simulink model "our_ch47"  (R2021a)
settings: Solver=FixedStepAuto  StartTime=0.0  StopTime=10  FixedStep=0.001  RelTol=1e-3  AbsTol=1e-3  EnableMultiTasking=on
undefined symbols (not defined in the file or in its folder): DiscIntNeverNeededParam, e2b, envs, PID_Param1, pos1, pos2, pos3, pos4, pos_load, tandem, X, x0, Y, Z
libraries: sm_lib x88, nesl_utility x25
(part 5 of 6)

== system our_ch47/Subsystem/直升机2 PID control/姿态控制器/航向控制器H-A/Altitude_Controller ==
  YawD : Inport
  Yaw : Inport  Port=2
  Constant : Constant  Value=0  OutDataTypeStr=Inherit: Inherit via back propagation
  Controller : Subsystem
  Saturation : Saturate  UpperLimit=45  LowerLimit=-45
  Saturation1 : Saturate  UpperLimit=45  LowerLimit=-45
  Subtract : Sum  Inputs=+-
  YawRateD : Outport  VectorParamsAs1DForOutWhenUnconnected=off
  wires:
  YawD/1 -> Subtract/1
  Yaw/1 -> Subtract/2
  Constant/1 -> Controller/2(reset)
  Saturation/1 -> YawRateD/1
  Controller/1(u) -> Saturation/1
  Subtract/1 -> Saturation1/1
  Saturation1/1 -> Controller/1(err)

== system our_ch47/Subsystem/直升机3 PID control/位置控制器/侧向位置控制器/侧向位置控制器 ==
  yd_m : Inport
  y_m : Inport  Port=2
  Constant : Constant  Value=0  OutDataTypeStr=Inherit: Inherit via back propagation
  PID_Controller : Subsystem
  Saturation : Saturate  UpperLimit=10  LowerLimit=-10
  Saturation1 : Saturate  UpperLimit=10  LowerLimit=-10
  Subtract : Sum  Inputs=+-
  VyD : Outport  VectorParamsAs1DForOutWhenUnconnected=off
  wires:
  yd_m/1 -> Subtract/1
  y_m/1 -> Subtract/2
  Constant/1 -> PID_Controller/2(reset)
  Saturation/1 -> VyD/1
  PID_Controller/1(u) -> Saturation/1
  Subtract/1 -> Saturation1/1
  Saturation1/1 -> PID_Controller/1(err)

== system our_ch47/Subsystem/直升机3 PID control/位置控制器/侧向速度控制器/PID_Controller ==
  err : Inport
  reset : Inport  Port=2
  Add : Sum
  I_Control : Subsystem  mask{ki=PID_Param1.Ki_Vy, max_i=0.3, min_i=-0.3}
  P_Control : Subsystem  mask{kp=PID_Param1.Kp_Vy}
  u : Outport  VectorParamsAs1DForOutWhenUnconnected=off
  wires:
  err/1 -> P_Control/1(err), I_Control/1(err)
  reset/1 -> I_Control/2(reset)
  P_Control/1(p_out) -> Add/1
  I_Control/1(i_out) -> Add/2
  Add/1 -> u/1

== system our_ch47/Subsystem/直升机3 PID control/位置控制器/前向位置控制器/前向位置控制器 ==
  xd_m : Inport
  x_m : Inport  Port=2
  Constant : Constant  Value=0  OutDataTypeStr=Inherit: Inherit via back propagation
  PID_Controller : Subsystem
  Saturation : Saturate  UpperLimit=12  LowerLimit=-12
  Saturation1 : Saturate  UpperLimit=10  LowerLimit=-10
  Subtract : Sum  Inputs=+-
  VxD : Outport  VectorParamsAs1DForOutWhenUnconnected=off
  wires:
  Saturation1/1 -> PID_Controller/1(err)
  Subtract/1 -> Saturation1/1
  PID_Controller/1(u) -> Saturation/1
  Saturation/1 -> VxD/1
  Constant/1 -> PID_Controller/2(reset)
  x_m/1 -> Subtract/2
  xd_m/1 -> Subtract/1

== system our_ch47/Subsystem/直升机3 PID control/位置控制器/前向速度控制器/PID_Controller ==
  err : Inport
  reset : Inport  Port=2
  Add : Sum
  I_Control : Subsystem  mask{ki=PID_Param1.Ki_Vx, max_i=0.3, min_i=-0.3}
  P_Control : Subsystem  mask{kp=PID_Param1.Kp_Vx}
  u : Outport  VectorParamsAs1DForOutWhenUnconnected=off
  wires:
  Add/1 -> u/1
  I_Control/1(i_out) -> Add/2
  P_Control/1(p_out) -> Add/1
  reset/1 -> I_Control/2(reset)
  err/1 -> I_Control/1(err), P_Control/1(err)

== system our_ch47/Subsystem/直升机3 PID control/位置控制器/垂向速度控制器/PID_Controller ==
  err : Inport
  reset : Inport  Port=2
  Add : Sum
  I_Control : Subsystem  mask{ki=PID_Param1.Ki_Vz, max_i=0.3, min_i=-0.3}
  P_Control : Subsystem  mask{kp=PID_Param1.Kp_Vz}
  u : Outport  VectorParamsAs1DForOutWhenUnconnected=off
  wires:
  Add/1 -> u/1
  I_Control/1(i_out) -> Add/2
  P_Control/1(p_out) -> Add/1
  reset/1 -> I_Control/2(reset)
  err/1 -> I_Control/1(err), P_Control/1(err)

== system our_ch47/Subsystem/直升机3 PID control/位置控制器/高度控制器/高度控制器H-A ==
  altitude_sp_m : Inport
  altitude_m : Inport  Port=2
  Constant : Constant  Value=0  OutDataTypeStr=Inherit: Inherit via back propagation
  PID_Controller : Subsystem
  Saturation : Saturate  UpperLimit=2  LowerLimit=-2
  Saturation1 : Saturate  UpperLimit=10  LowerLimit=-10
  Subtract : Sum  Inputs=+-
  VzD : Outport  VectorParamsAs1DForOutWhenUnconnected=off
  wires:
  Saturation1/1 -> PID_Controller/1(err)
  Subtract/1 -> Saturation1/1
  PID_Controller/1(u) -> Saturation/1
  Saturation/1 -> VzD/1
  Constant/1 -> PID_Controller/2(reset)
  altitude_m/1 -> Subtract/2
  altitude_sp_m/1 -> Subtract/1

== system our_ch47/Subsystem/直升机3 PID control/姿态控制器/俯仰控制器H-A/AltitudeV_Controller ==
  PitchRateD : Inport
  PitchRate : Inport  Port=2
  PID_Controller : Subsystem
  Saturation : Saturate  UpperLimit=5  LowerLimit=-5
  Subtract : Sum  Inputs=+-
  Lon : Outport  VectorParamsAs1DForOutWhenUnconnected=off
  wires:
  PID_Controller/1(u) -> Saturation/1
  Saturation/1 -> Lon/1
  Subtract/1 -> PID_Controller/1(err)
  PitchRate/1 -> Subtract/2
  PitchRateD/1 -> Subtract/1

== system our_ch47/Subsystem/直升机3 PID control/姿态控制器/俯仰控制器H-A/角度换 ==
  PitchD : Inport
  Pitch : Inport  Port=2
  PID_Controller : Subsystem
  Saturation : Saturate  UpperLimit=45  LowerLimit=-45
  Saturation1 : Saturate  UpperLimit=45  LowerLimit=-45
  Subtract : Sum  Inputs=+-
  PitchRateD : Outport  VectorParamsAs1DForOutWhenUnconnected=off
  wires:
  Saturation/1 -> PitchRateD/1
  Subtract/1 -> Saturation1/1
  Saturation1/1 -> PID_Controller/1(err)
  PID_Controller/1(u) -> Saturation/1
  Pitch/1 -> Subtract/2
  PitchD/1 -> Subtract/1

== system our_ch47/Subsystem/直升机3 PID control/姿态控制器/滚转控制器H-A/AltitudeV_Controller ==
  RollRateD : Inport
  RollRate : Inport  Port=2
  Constant : Constant  Value=0  OutDataTypeStr=Inherit: Inherit via back propagation
  PID_Controller : Subsystem
  Saturation : Saturate  UpperLimit=5  LowerLimit=-5
  Subtract : Sum  Inputs=+-
  Lat : Outport  VectorParamsAs1DForOutWhenUnconnected=off
  wires:
  PID_Controller/1(u) -> Saturation/1
  Saturation/1 -> Lat/1
  Constant/1 -> PID_Controller/2(reset)
  Subtract/1 -> PID_Controller/1(err)
  RollRate/1 -> Subtract/2
  RollRateD/1 -> Subtract/1

== system our_ch47/Subsystem/直升机3 PID control/姿态控制器/滚转控制器H-A/Altitude_Controller ==
  RollD : Inport
  Roll : Inport  Port=2
  PID_Controller : Subsystem
  Saturation : Saturate  UpperLimit=45  LowerLimit=-45
  Saturation1 : Saturate  UpperLimit=45  LowerLimit=-45
  Subtract : Sum  Inputs=+-
  RollRateD : Outport  VectorParamsAs1DForOutWhenUnconnected=off
  wires:
  Saturation1/1 -> PID_Controller/1(err)
  Subtract/1 -> Saturation1/1
  PID_Controller/1(u) -> Saturation/1
  Saturation/1 -> RollRateD/1
  Roll/1 -> Subtract/2
  RollD/1 -> Subtract/1

== system our_ch47/Subsystem/直升机3 PID control/姿态控制器/航向控制器H-A/AltitudeV_Controller ==
  YawRateD : Inport
  YawRate : Inport  Port=2
  Constant : Constant  Value=0  OutDataTypeStr=Inherit: Inherit via back propagation
  Controller : Subsystem
  Saturation : Saturate  UpperLimit=5  LowerLimit=-5
  Subtract : Sum  Inputs=+-
  Ped : Outport  VectorParamsAs1DForOutWhenUnconnected=off
  wires:
  Controller/1(u) -> Saturation/1
  Saturation/1 -> Ped/1
  Constant/1 -> Controller/2(reset)
  Subtract/1 -> Controller/1(err)
  YawRate/1 -> Subtract/2
  YawRateD/1 -> Subtract/1

== system our_ch47/Subsystem/直升机3 PID control/姿态控制器/航向控制器H-A/Altitude_Controller ==
  YawD : Inport
  Yaw : Inport  Port=2
  Constant : Constant  Value=0  OutDataTypeStr=Inherit: Inherit via back propagation
  Controller : Subsystem
  Saturation : Saturate  UpperLimit=45  LowerLimit=-45
  Saturation1 : Saturate  UpperLimit=45  LowerLimit=-45
  Subtract : Sum  Inputs=+-
  YawRateD : Outport  VectorParamsAs1DForOutWhenUnconnected=off
  wires:
  Saturation1/1 -> Controller/1(err)
  Subtract/1 -> Saturation1/1
  Controller/1(u) -> Saturation/1
  Saturation/1 -> YawRateD/1
  Constant/1 -> Controller/2(reset)
  Yaw/1 -> Subtract/2
  YawD/1 -> Subtract/1

== system our_ch47/Subsystem/直升机4 PID control/位置控制器/侧向位置控制器/侧向位置控制器 ==
  yd_m : Inport
  y_m : Inport  Port=2
  Constant : Constant  Value=0  OutDataTypeStr=Inherit: Inherit via back propagation
  PID_Controller : Subsystem
  Saturation : Saturate  UpperLimit=10  LowerLimit=-10
  Saturation1 : Saturate  UpperLimit=10  LowerLimit=-10
  Subtract : Sum  Inputs=+-
  VyD : Outport  VectorParamsAs1DForOutWhenUnconnected=off
  wires:
  Saturation1/1 -> PID_Controller/1(err)
  Subtract/1 -> Saturation1/1
  PID_Controller/1(u) -> Saturation/1
  Saturation/1 -> VyD/1
  Constant/1 -> PID_Controller/2(reset)
  y_m/1 -> Subtract/2
  yd_m/1 -> Subtract/1

== system our_ch47/Subsystem/直升机4 PID control/位置控制器/侧向速度控制器/PID_Controller ==
  err : Inport
  reset : Inport  Port=2
  Add : Sum
  I_Control : Subsystem  mask{ki=PID_Param1.Ki_Vy, max_i=0.3, min_i=-0.3}
  P_Control : Subsystem  mask{kp=PID_Param1.Kp_Vy}
  u : Outport  VectorParamsAs1DForOutWhenUnconnected=off
  wires:
  Add/1 -> u/1
  I_Control/1(i_out) -> Add/2
  P_Control/1(p_out) -> Add/1
  reset/1 -> I_Control/2(reset)
  err/1 -> I_Control/1(err), P_Control/1(err)

== system our_ch47/Subsystem/直升机4 PID control/位置控制器/前向位置控制器/前向位置控制器 ==
  xd_m : Inport
  x_m : Inport  Port=2
  Constant : Constant  Value=0  OutDataTypeStr=Inherit: Inherit via back propagation
  PID_Controller : Subsystem
  Saturation : Saturate  UpperLimit=12  LowerLimit=-12
  Saturation1 : Saturate  UpperLimit=10  LowerLimit=-10
  Subtract : Sum  Inputs=+-
  VxD : Outport  VectorParamsAs1DForOutWhenUnconnected=off
  wires:
  xd_m/1 -> Subtract/1
  x_m/1 -> Subtract/2
  Constant/1 -> PID_Controller/2(reset)
  Saturation/1 -> VxD/1
  PID_Controller/1(u) -> Saturation/1
  Subtract/1 -> Saturation1/1
  Saturation1/1 -> PID_Controller/1(err)

== system our_ch47/Subsystem/直升机4 PID control/位置控制器/前向速度控制器/PID_Controller ==
  err : Inport
  reset : Inport  Port=2
  Add : Sum
  I_Control : Subsystem  mask{ki=PID_Param1.Ki_Vx, max_i=0.3, min_i=-0.3}
  P_Control : Subsystem  mask{kp=PID_Param1.Kp_Vx}
  u : Outport  VectorParamsAs1DForOutWhenUnconnected=off
  wires:
  err/1 -> P_Control/1(err), I_Control/1(err)
  reset/1 -> I_Control/2(reset)
  P_Control/1(p_out) -> Add/1
  I_Control/1(i_out) -> Add/2
  Add/1 -> u/1

== system our_ch47/Subsystem/直升机4 PID control/位置控制器/垂向速度控制器/PID_Controller ==
  err : Inport
  reset : Inport  Port=2
  Add : Sum
  I_Control : Subsystem  mask{ki=PID_Param1.Ki_Vz, max_i=0.3, min_i=-0.3}
  P_Control : Subsystem  mask{kp=PID_Param1.Kp_Vz}
  u : Outport  VectorParamsAs1DForOutWhenUnconnected=off
  wires:
  err/1 -> P_Control/1(err), I_Control/1(err)
  reset/1 -> I_Control/2(reset)
  P_Control/1(p_out) -> Add/1
  I_Control/1(i_out) -> Add/2
  Add/1 -> u/1

== system our_ch47/Subsystem/直升机4 PID control/位置控制器/高度控制器/高度控制器H-A ==
  altitude_sp_m : Inport
  altitude_m : Inport  Port=2
  Constant : Constant  Value=0  OutDataTypeStr=Inherit: Inherit via back propagation
  PID_Controller : Subsystem
  Saturation : Saturate  UpperLimit=2  LowerLimit=-2
  Saturation1 : Saturate  UpperLimit=10  LowerLimit=-10
  Subtract : Sum  Inputs=+-
  VzD : Outport  VectorParamsAs1DForOutWhenUnconnected=off
  wires:
  altitude_sp_m/1 -> Subtract/1
  altitude_m/1 -> Subtract/2
  Constant/1 -> PID_Controller/2(reset)
  Saturation/1 -> VzD/1
  PID_Controller/1(u) -> Saturation/1
  Subtract/1 -> Saturation1/1
  Saturation1/1 -> PID_Controller/1(err)

== system our_ch47/Subsystem/直升机4 PID control/姿态控制器/俯仰控制器H-A/AltitudeV_Controller ==
  PitchRateD : Inport
  PitchRate : Inport  Port=2
  PID_Controller : Subsystem
  Saturation : Saturate  UpperLimit=5  LowerLimit=-5
  Subtract : Sum  Inputs=+-
  Lon : Outport  VectorParamsAs1DForOutWhenUnconnected=off
  wires:
  PitchRateD/1 -> Subtract/1
  PitchRate/1 -> Subtract/2
  Subtract/1 -> PID_Controller/1(err)
  Saturation/1 -> Lon/1
  PID_Controller/1(u) -> Saturation/1

== system our_ch47/Subsystem/直升机4 PID control/姿态控制器/俯仰控制器H-A/角度换 ==
  PitchD : Inport
  Pitch : Inport  Port=2
  PID_Controller : Subsystem
  Saturation : Saturate  UpperLimit=45  LowerLimit=-45
  Saturation1 : Saturate  UpperLimit=45  LowerLimit=-45
  Subtract : Sum  Inputs=+-
  PitchRateD : Outport  VectorParamsAs1DForOutWhenUnconnected=off
  wires:
  PitchD/1 -> Subtract/1
  Pitch/1 -> Subtract/2
  PID_Controller/1(u) -> Saturation/1
  Saturation1/1 -> PID_Controller/1(err)
  Subtract/1 -> Saturation1/1
  Saturation/1 -> PitchRateD/1

== system our_ch47/Subsystem/直升机4 PID control/姿态控制器/滚转控制器H-A/AltitudeV_Controller ==
  RollRateD : Inport
  RollRate : Inport  Port=2
  Constant : Constant  Value=0  OutDataTypeStr=Inherit: Inherit via back propagation
  PID_Controller : Subsystem
  Saturation : Saturate  UpperLimit=5  LowerLimit=-5
  Subtract : Sum  Inputs=+-
  Lat : Outport  VectorParamsAs1DForOutWhenUnconnected=off
  wires:
  RollRateD/1 -> Subtract/1
  RollRate/1 -> Subtract/2
  Subtract/1 -> PID_Controller/1(err)
  Constant/1 -> PID_Controller/2(reset)
  Saturation/1 -> Lat/1
  PID_Controller/1(u) -> Saturation/1

== system our_ch47/Subsystem/直升机4 PID control/姿态控制器/滚转控制器H-A/Altitude_Controller ==
  RollD : Inport
  Roll : Inport  Port=2
  PID_Controller : Subsystem
  Saturation : Saturate  UpperLimit=45  LowerLimit=-45
  Saturation1 : Saturate  UpperLimit=45  LowerLimit=-45
  Subtract : Sum  Inputs=+-
  RollRateD : Outport  VectorParamsAs1DForOutWhenUnconnected=off
  wires:
  RollD/1 -> Subtract/1
  Roll/1 -> Subtract/2
  Saturation/1 -> RollRateD/1
  PID_Controller/1(u) -> Saturation/1
  Subtract/1 -> Saturation1/1
  Saturation1/1 -> PID_Controller/1(err)

== system our_ch47/Subsystem/直升机4 PID control/姿态控制器/航向控制器H-A/AltitudeV_Controller ==
  YawRateD : Inport
  YawRate : Inport  Port=2
  Constant : Constant  Value=0  OutDataTypeStr=Inherit: Inherit via back propagation
  Controller : Subsystem
  Saturation : Saturate  UpperLimit=5  LowerLimit=-5
  Subtract : Sum  Inputs=+-
  Ped : Outport  VectorParamsAs1DForOutWhenUnconnected=off
  wires:
  YawRateD/1 -> Subtract/1
  YawRate/1 -> Subtract/2
  Subtract/1 -> Controller/1(err)
  Constant/1 -> Controller/2(reset)
  Saturation/1 -> Ped/1
  Controller/1(u) -> Saturation/1

== system our_ch47/Subsystem/直升机4 PID control/姿态控制器/航向控制器H-A/Altitude_Controller ==
  YawD : Inport
  Yaw : Inport  Port=2
  Constant : Constant  Value=0  OutDataTypeStr=Inherit: Inherit via back propagation
  Controller : Subsystem
  Saturation : Saturate  UpperLimit=45  LowerLimit=-45
  Saturation1 : Saturate  UpperLimit=45  LowerLimit=-45
  Subtract : Sum  Inputs=+-
  YawRateD : Outport  VectorParamsAs1DForOutWhenUnconnected=off
  wires:
  YawD/1 -> Subtract/1
  Yaw/1 -> Subtract/2
  Constant/1 -> Controller/2(reset)
  Saturation/1 -> YawRateD/1
  Controller/1(u) -> Saturation/1
  Subtract/1 -> Saturation1/1
  Saturation1/1 -> Controller/1(err)

== system our_ch47/Subsystem/直升机1 PID control/位置控制器/侧向位置控制器/侧向位置控制器/PID_Controller ==
  err : Inport
  reset : Inport  Port=2
  Add : Sum
  I_Control : Subsystem  mask{ki=PID_Param1.Ki_y, max_i=1, min_i=-1}
  P_Control : Subsystem  mask{kp=PID_Param1.Kp_y}
  u : Outport  VectorParamsAs1DForOutWhenUnconnected=off
  wires:
  Add/1 -> u/1
  I_Control/1(i_out) -> Add/2
  P_Control/1(p_out) -> Add/1
  reset/1 -> I_Control/2(reset)
  err/1 -> I_Control/1(err), P_Control/1(err)

== system our_ch47/Subsystem/直升机1 PID control/位置控制器/侧向速度控制器/PID_Controller/I_Control ==
  err : Inport
  reset : Inport  Port=2
  Constant : Constant  Value=0  OutDataTypeStr=single
  Discrete-Time Integrator : DiscreteIntegrator  ExternalReset=level  InitialConditionSource=external  SampleTime=-1  ICPrevOutput=DiscIntNeverNeededParam  ICPrevScaledInput=DiscIntNeverNeededParam
  Multiply : Product  OutDataTypeStr=Inherit: Same as first input
  Saturation : Saturate  UpperLimit=max_i  LowerLimit=min_i
  ki : Constant  Value=ki  OutDataTypeStr=single
  i_out : Outport  VectorParamsAs1DForOutWhenUnconnected=off
  wires:
  ki/1 -> Multiply/1
  Saturation/1 -> i_out/1
  Discrete-Time Integrator/1 -> Saturation/1
  Constant/1 -> Discrete-Time Integrator/3
  reset/1 -> Discrete-Time Integrator/2
  Multiply/1 -> Discrete-Time Integrator/1
  err/1 -> Multiply/2

== system our_ch47/Subsystem/直升机1 PID control/位置控制器/侧向速度控制器/PID_Controller/P_Control ==
  err : Inport
  Multiply : Product  OutDataTypeStr=Inherit: Same as first input
  kp : Constant  Value=kp  OutDataTypeStr=single
  p_out : Outport  VectorParamsAs1DForOutWhenUnconnected=off
  wires:
  Multiply/1 -> p_out/1
  kp/1 -> Multiply/1
  err/1 -> Multiply/2

== system our_ch47/Subsystem/直升机1 PID control/位置控制器/前向位置控制器/前向位置控制器/PID_Controller ==
  err : Inport
  reset : Inport  Port=2
  Add : Sum
  I_Control : Subsystem  mask{ki=PID_Param1.Ki_x, max_i=1, min_i=-1}
  P_Control : Subsystem  mask{kp=PID_Param1.Kp_x}
  u : Outport  VectorParamsAs1DForOutWhenUnconnected=off
  wires:
  err/1 -> P_Control/1(err), I_Control/1(err)
  reset/1 -> I_Control/2(reset)
  P_Control/1(p_out) -> Add/1
  I_Control/1(i_out) -> Add/2
  Add/1 -> u/1

== system our_ch47/Subsystem/直升机1 PID control/位置控制器/前向速度控制器/PID_Controller/I_Control ==
  err : Inport
  reset : Inport  Port=2
  Constant : Constant  Value=0  OutDataTypeStr=single
  Discrete-Time Integrator : DiscreteIntegrator  ExternalReset=level  InitialConditionSource=external  SampleTime=-1  ICPrevOutput=DiscIntNeverNeededParam  ICPrevScaledInput=DiscIntNeverNeededParam
  Multiply : Product  OutDataTypeStr=Inherit: Same as first input
  Saturation : Saturate  UpperLimit=max_i  LowerLimit=min_i
  ki : Constant  Value=ki  OutDataTypeStr=single
  i_out : Outport  VectorParamsAs1DForOutWhenUnconnected=off
  wires:
  err/1 -> Multiply/2
  Multiply/1 -> Discrete-Time Integrator/1
  reset/1 -> Discrete-Time Integrator/2
  Constant/1 -> Discrete-Time Integrator/3
  Discrete-Time Integrator/1 -> Saturation/1
  Saturation/1 -> i_out/1
  ki/1 -> Multiply/1

== system our_ch47/Subsystem/直升机1 PID control/位置控制器/前向速度控制器/PID_Controller/P_Control ==
  err : Inport
  Multiply : Product  OutDataTypeStr=Inherit: Same as first input
  kp : Constant  Value=kp  OutDataTypeStr=single
  p_out : Outport  VectorParamsAs1DForOutWhenUnconnected=off
  wires:
  err/1 -> Multiply/2
  kp/1 -> Multiply/1
  Multiply/1 -> p_out/1

== system our_ch47/Subsystem/直升机1 PID control/位置控制器/垂向速度控制器/PID_Controller/I_Control ==
  err : Inport
  reset : Inport  Port=2
  Constant : Constant  Value=0  OutDataTypeStr=single
  Discrete-Time Integrator : DiscreteIntegrator  ExternalReset=level  InitialConditionSource=external  SampleTime=-1  ICPrevOutput=DiscIntNeverNeededParam  ICPrevScaledInput=DiscIntNeverNeededParam
  Multiply : Product  OutDataTypeStr=Inherit: Same as first input
  Saturation : Saturate  UpperLimit=max_i  LowerLimit=min_i
  ki : Constant  Value=ki  OutDataTypeStr=single
  i_out : Outport  VectorParamsAs1DForOutWhenUnconnected=off
  wires:
  err/1 -> Multiply/2
  Multiply/1 -> Discrete-Time Integrator/1
  reset/1 -> Discrete-Time Integrator/2
  Constant/1 -> Discrete-Time Integrator/3
  Discrete-Time Integrator/1 -> Saturation/1
  Saturation/1 -> i_out/1
  ki/1 -> Multiply/1

== system our_ch47/Subsystem/直升机1 PID control/位置控制器/垂向速度控制器/PID_Controller/P_Control ==
  err : Inport
  Multiply : Product  OutDataTypeStr=Inherit: Same as first input
  kp : Constant  Value=kp  OutDataTypeStr=single
  p_out : Outport  VectorParamsAs1DForOutWhenUnconnected=off
  wires:
  err/1 -> Multiply/2
  kp/1 -> Multiply/1
  Multiply/1 -> p_out/1

== system our_ch47/Subsystem/直升机1 PID control/位置控制器/高度控制器/高度控制器H-A/PID_Controller ==
  err : Inport
  reset : Inport  Port=2
  Add : Sum
  I_Control : Subsystem  mask{ki=PID_Param1.Ki_Hight, max_i=1, min_i=-1}
  P_Control : Subsystem  mask{kp=PID_Param1.Kp_Hight}
  u : Outport  VectorParamsAs1DForOutWhenUnconnected=off
  wires:
  err/1 -> P_Control/1(err), I_Control/1(err)
  reset/1 -> I_Control/2(reset)
  P_Control/1(p_out) -> Add/1
  I_Control/1(i_out) -> Add/2
  Add/1 -> u/1

== system our_ch47/Subsystem/直升机1 PID control/姿态控制器/俯仰控制器H-A/AltitudeV_Controller/PID_Controller ==
  err : Inport
  Add : Sum
  I_Control : Subsystem  mask{ki=PID_Param1.Ki_pitchrate, max_i=0.3, min_i=-0.3}
  P_Control : Subsystem  mask{kp=PID_Param1.Kp_pitchrate}
  u : Outport  VectorParamsAs1DForOutWhenUnconnected=off
  wires:
  err/1 -> P_Control/1(err), I_Control/1(err)
  P_Control/1(p_out) -> Add/1
  I_Control/1(i_out) -> Add/2
  Add/1 -> u/1

== system our_ch47/Subsystem/直升机1 PID control/姿态控制器/俯仰控制器H-A/角度换/PID_Controller ==
  err : Inport
  Add : Sum
  I_Control : Subsystem  mask{ki=PID_Param1.Ki_pitch, max_i=0.3, min_i=-0.3}
  P_Control : Subsystem  mask{kp=PID_Param1.Kp_pitch}
  u : Outport  VectorParamsAs1DForOutWhenUnconnected=off
  wires:
  err/1 -> P_Control/1(err), I_Control/1(err)
  P_Control/1(p_out) -> Add/1
  I_Control/1(i_out) -> Add/2
  Add/1 -> u/1

== system our_ch47/Subsystem/直升机1 PID control/姿态控制器/滚转控制器H-A/AltitudeV_Controller/PID_Controller ==
  err : Inport
  reset : Inport  Port=2
  Add : Sum
  I_Control : Subsystem  mask{ki=PID_Param1.Ki_rollrate, max_i=0.3, min_i=-0.3}
  P_Control : Subsystem  mask{kp=PID_Param1.Kp_rollrate}
  u : Outport  VectorParamsAs1DForOutWhenUnconnected=off
  wires:
  err/1 -> P_Control/1(err), I_Control/1(err)
  reset/1 -> I_Control/2(reset)
  P_Control/1(p_out) -> Add/1  "p_out"
  I_Control/1(i_out) -> Add/2  "i_out"
  Add/1 -> u/1

== system our_ch47/Subsystem/直升机1 PID control/姿态控制器/滚转控制器H-A/Altitude_Controller/PID_Controller ==
  err : Inport
  Add : Sum
  Constant : Constant  Value=0
  I_Control : Subsystem  mask{ki=PID_Param1.Ki_roll, max_i=0.3, min_i=-0.3}
  P_Control : Subsystem  mask{kp=PID_Param1.Kp_roll}
  u : Outport  VectorParamsAs1DForOutWhenUnconnected=off
  wires:
  err/1 -> P_Control/1(err), I_Control/1(err)
  P_Control/1(p_out) -> Add/1
  I_Control/1(i_out) -> Add/2
  Add/1 -> u/1
  Constant/1 -> I_Control/2(reset)

== system our_ch47/Subsystem/直升机1 PID control/姿态控制器/航向控制器H-A/AltitudeV_Controller/Controller ==
  err : Inport
  reset : Inport  Port=2
  Add : Sum
  I_Control : Subsystem  mask{ki=PID_Param1.Ki_yawrate, max_i=0.3, min_i=-0.3}
  P_Control : Subsystem  mask{kp=PID_Param1.Kp_yawrate}
  u : Outport  VectorParamsAs1DForOutWhenUnconnected=off
  wires:
  err/1 -> P_Control/1(err), I_Control/1(err)
  reset/1 -> I_Control/2(reset)
  P_Control/1(p_out) -> Add/1
  I_Control/1(i_out) -> Add/2
  Add/1 -> u/1

== system our_ch47/Subsystem/直升机1 PID control/姿态控制器/航向控制器H-A/Altitude_Controller/Controller ==
  err : Inport
  reset : Inport  Port=2
  Add : Sum
  I_Control : Subsystem  mask{ki=PID_Param1.Ki_yaw, max_i=5, min_i=-5}
  P_Control : Subsystem  mask{kp=PID_Param1.Kp_yaw}
  u : Outport  VectorParamsAs1DForOutWhenUnconnected=off
  wires:
  err/1 -> P_Control/1(err), I_Control/1(err)
  reset/1 -> I_Control/2(reset)
  P_Control/1(p_out) -> Add/1
  I_Control/1(i_out) -> Add/2
  Add/1 -> u/1

== system our_ch47/Subsystem/直升机2 PID control/位置控制器/侧向位置控制器/侧向位置控制器/PID_Controller ==
  err : Inport
  reset : Inport  Port=2
  Add : Sum
  I_Control : Subsystem  mask{ki=PID_Param1.Ki_y, max_i=1, min_i=-1}
  P_Control : Subsystem  mask{kp=PID_Param1.Kp_y}
  u : Outport  VectorParamsAs1DForOutWhenUnconnected=off
  wires:
  Add/1 -> u/1
  I_Control/1(i_out) -> Add/2
  P_Control/1(p_out) -> Add/1
  reset/1 -> I_Control/2(reset)
  err/1 -> I_Control/1(err), P_Control/1(err)

== system our_ch47/Subsystem/直升机2 PID control/位置控制器/侧向速度控制器/PID_Controller/I_Control ==
  err : Inport
  reset : Inport  Port=2
  Constant : Constant  Value=0  OutDataTypeStr=single
  Discrete-Time Integrator : DiscreteIntegrator  ExternalReset=level  InitialConditionSource=external  SampleTime=-1  ICPrevOutput=DiscIntNeverNeededParam  ICPrevScaledInput=DiscIntNeverNeededParam
  Multiply : Product  OutDataTypeStr=Inherit: Same as first input
  Saturation : Saturate  UpperLimit=max_i  LowerLimit=min_i
  ki : Constant  Value=ki  OutDataTypeStr=single
  i_out : Outport  VectorParamsAs1DForOutWhenUnconnected=off
  wires:
  ki/1 -> Multiply/1
  Saturation/1 -> i_out/1
  Discrete-Time Integrator/1 -> Saturation/1
  Constant/1 -> Discrete-Time Integrator/3
  reset/1 -> Discrete-Time Integrator/2
  Multiply/1 -> Discrete-Time Integrator/1
  err/1 -> Multiply/2

== system our_ch47/Subsystem/直升机2 PID control/位置控制器/侧向速度控制器/PID_Controller/P_Control ==
  err : Inport
  Multiply : Product  OutDataTypeStr=Inherit: Same as first input
  kp : Constant  Value=kp  OutDataTypeStr=single
  p_out : Outport  VectorParamsAs1DForOutWhenUnconnected=off
  wires:
  Multiply/1 -> p_out/1
  kp/1 -> Multiply/1
  err/1 -> Multiply/2

== system our_ch47/Subsystem/直升机2 PID control/位置控制器/前向位置控制器/前向位置控制器/PID_Controller ==
  err : Inport
  reset : Inport  Port=2
  Add : Sum
  I_Control : Subsystem  mask{ki=PID_Param1.Ki_x, max_i=1, min_i=-1}
  P_Control : Subsystem  mask{kp=PID_Param1.Kp_x}
  u : Outport  VectorParamsAs1DForOutWhenUnconnected=off
  wires:
  err/1 -> P_Control/1(err), I_Control/1(err)
  reset/1 -> I_Control/2(reset)
  P_Control/1(p_out) -> Add/1
  I_Control/1(i_out) -> Add/2
  Add/1 -> u/1

== system our_ch47/Subsystem/直升机2 PID control/位置控制器/前向速度控制器/PID_Controller/I_Control ==
  err : Inport
  reset : Inport  Port=2
  Constant : Constant  Value=0  OutDataTypeStr=single
  Discrete-Time Integrator : DiscreteIntegrator  ExternalReset=level  InitialConditionSource=external  SampleTime=-1  ICPrevOutput=DiscIntNeverNeededParam  ICPrevScaledInput=DiscIntNeverNeededParam
  Multiply : Product  OutDataTypeStr=Inherit: Same as first input
  Saturation : Saturate  UpperLimit=max_i  LowerLimit=min_i
  ki : Constant  Value=ki  OutDataTypeStr=single
  i_out : Outport  VectorParamsAs1DForOutWhenUnconnected=off
  wires:
  err/1 -> Multiply/2
  Multiply/1 -> Discrete-Time Integrator/1
  reset/1 -> Discrete-Time Integrator/2
  Constant/1 -> Discrete-Time Integrator/3
  Discrete-Time Integrator/1 -> Saturation/1
  Saturation/1 -> i_out/1
  ki/1 -> Multiply/1

== system our_ch47/Subsystem/直升机2 PID control/位置控制器/前向速度控制器/PID_Controller/P_Control ==
  err : Inport
  Multiply : Product  OutDataTypeStr=Inherit: Same as first input
  kp : Constant  Value=kp  OutDataTypeStr=single
  p_out : Outport  VectorParamsAs1DForOutWhenUnconnected=off
  wires:
  err/1 -> Multiply/2
  kp/1 -> Multiply/1
  Multiply/1 -> p_out/1

== system our_ch47/Subsystem/直升机2 PID control/位置控制器/垂向速度控制器/PID_Controller/I_Control ==
  err : Inport
  reset : Inport  Port=2
  Constant : Constant  Value=0  OutDataTypeStr=single
  Discrete-Time Integrator : DiscreteIntegrator  ExternalReset=level  InitialConditionSource=external  SampleTime=-1  ICPrevOutput=DiscIntNeverNeededParam  ICPrevScaledInput=DiscIntNeverNeededParam
  Multiply : Product  OutDataTypeStr=Inherit: Same as first input
  Saturation : Saturate  UpperLimit=max_i  LowerLimit=min_i
  ki : Constant  Value=ki  OutDataTypeStr=single
  i_out : Outport  VectorParamsAs1DForOutWhenUnconnected=off
  wires:
  err/1 -> Multiply/2
  Multiply/1 -> Discrete-Time Integrator/1
  reset/1 -> Discrete-Time Integrator/2
  Constant/1 -> Discrete-Time Integrator/3
  Discrete-Time Integrator/1 -> Saturation/1
  Saturation/1 -> i_out/1
  ki/1 -> Multiply/1

== system our_ch47/Subsystem/直升机2 PID control/位置控制器/垂向速度控制器/PID_Controller/P_Control ==
  err : Inport
  Multiply : Product  OutDataTypeStr=Inherit: Same as first input
  kp : Constant  Value=kp  OutDataTypeStr=single
  p_out : Outport  VectorParamsAs1DForOutWhenUnconnected=off
  wires:
  err/1 -> Multiply/2
  kp/1 -> Multiply/1
  Multiply/1 -> p_out/1

== system our_ch47/Subsystem/直升机2 PID control/位置控制器/高度控制器/高度控制器H-A/PID_Controller ==
  err : Inport
  reset : Inport  Port=2
  Add : Sum
  I_Control : Subsystem  mask{ki=PID_Param1.Ki_Hight, max_i=1, min_i=-1}
  P_Control : Subsystem  mask{kp=PID_Param1.Kp_Hight}
  u : Outport  VectorParamsAs1DForOutWhenUnconnected=off
  wires:
  err/1 -> P_Control/1(err), I_Control/1(err)
  reset/1 -> I_Control/2(reset)
  P_Control/1(p_out) -> Add/1
  I_Control/1(i_out) -> Add/2
  Add/1 -> u/1

== system our_ch47/Subsystem/直升机2 PID control/姿态控制器/俯仰控制器H-A/AltitudeV_Controller/PID_Controller ==
  err : Inport
  Add : Sum
  I_Control : Subsystem  mask{ki=PID_Param1.Ki_pitchrate, max_i=0.3, min_i=-0.3}
  P_Control : Subsystem  mask{kp=PID_Param1.Kp_pitchrate}
  u : Outport  VectorParamsAs1DForOutWhenUnconnected=off
  wires:
  err/1 -> P_Control/1(err), I_Control/1(err)
  P_Control/1(p_out) -> Add/1
  I_Control/1(i_out) -> Add/2
  Add/1 -> u/1

== system our_ch47/Subsystem/直升机2 PID control/姿态控制器/俯仰控制器H-A/角度换/PID_Controller ==
  err : Inport
  Add : Sum
  I_Control : Subsystem  mask{ki=PID_Param1.Ki_pitch, max_i=0.3, min_i=-0.3}
  P_Control : Subsystem  mask{kp=PID_Param1.Kp_pitch}
  u : Outport  VectorParamsAs1DForOutWhenUnconnected=off
  wires:
  err/1 -> P_Control/1(err), I_Control/1(err)
  P_Control/1(p_out) -> Add/1
  I_Control/1(i_out) -> Add/2
  Add/1 -> u/1

== system our_ch47/Subsystem/直升机2 PID control/姿态控制器/滚转控制器H-A/AltitudeV_Controller/PID_Controller ==
  err : Inport
  reset : Inport  Port=2
  Add : Sum
  I_Control : Subsystem  mask{ki=PID_Param1.Ki_rollrate, max_i=0.3, min_i=-0.3}
  P_Control : Subsystem  mask{kp=PID_Param1.Kp_rollrate}
  u : Outport  VectorParamsAs1DForOutWhenUnconnected=off
  wires:
  err/1 -> P_Control/1(err), I_Control/1(err)
  reset/1 -> I_Control/2(reset)
  P_Control/1(p_out) -> Add/1  "p_out"
  I_Control/1(i_out) -> Add/2  "i_out"
  Add/1 -> u/1

== system our_ch47/Subsystem/直升机2 PID control/姿态控制器/滚转控制器H-A/Altitude_Controller/PID_Controller ==
  err : Inport
  Add : Sum
  Constant : Constant  Value=0
  I_Control : Subsystem  mask{ki=PID_Param1.Ki_roll, max_i=0.3, min_i=-0.3}
  P_Control : Subsystem  mask{kp=PID_Param1.Kp_roll}
  u : Outport  VectorParamsAs1DForOutWhenUnconnected=off
  wires:
  err/1 -> P_Control/1(err), I_Control/1(err)
  P_Control/1(p_out) -> Add/1
  I_Control/1(i_out) -> Add/2
  Add/1 -> u/1
  Constant/1 -> I_Control/2(reset)

== system our_ch47/Subsystem/直升机2 PID control/姿态控制器/航向控制器H-A/AltitudeV_Controller/Controller ==
  err : Inport
  reset : Inport  Port=2
  Add : Sum
  I_Control : Subsystem  mask{ki=PID_Param1.Ki_yawrate, max_i=0.3, min_i=-0.3}
  P_Control : Subsystem  mask{kp=PID_Param1.Kp_yawrate}
  u : Outport  VectorParamsAs1DForOutWhenUnconnected=off
  wires:
  err/1 -> P_Control/1(err), I_Control/1(err)
  reset/1 -> I_Control/2(reset)
  P_Control/1(p_out) -> Add/1
  I_Control/1(i_out) -> Add/2
  Add/1 -> u/1

== system our_ch47/Subsystem/直升机2 PID control/姿态控制器/航向控制器H-A/Altitude_Controller/Controller ==
  err : Inport
  reset : Inport  Port=2
  Add : Sum
  I_Control : Subsystem  mask{ki=PID_Param1.Ki_yaw, max_i=5, min_i=-5}
  P_Control : Subsystem  mask{kp=PID_Param1.Kp_yaw}
  u : Outport  VectorParamsAs1DForOutWhenUnconnected=off
  wires:
  err/1 -> P_Control/1(err), I_Control/1(err)
  reset/1 -> I_Control/2(reset)
  P_Control/1(p_out) -> Add/1
  I_Control/1(i_out) -> Add/2
  Add/1 -> u/1

== system our_ch47/Subsystem/直升机3 PID control/位置控制器/侧向位置控制器/侧向位置控制器/PID_Controller ==
  err : Inport
  reset : Inport  Port=2
  Add : Sum
  I_Control : Subsystem  mask{ki=PID_Param1.Ki_y, max_i=1, min_i=-1}
  P_Control : Subsystem  mask{kp=PID_Param1.Kp_y}
  u : Outport  VectorParamsAs1DForOutWhenUnconnected=off
  wires:
  err/1 -> P_Control/1(err), I_Control/1(err)
  reset/1 -> I_Control/2(reset)
  P_Control/1(p_out) -> Add/1
  I_Control/1(i_out) -> Add/2
  Add/1 -> u/1

== system our_ch47/Subsystem/直升机3 PID control/位置控制器/侧向速度控制器/PID_Controller/I_Control ==
  err : Inport
  reset : Inport  Port=2
  Constant : Constant  Value=0  OutDataTypeStr=single
  Discrete-Time Integrator : DiscreteIntegrator  ExternalReset=level  InitialConditionSource=external  SampleTime=-1  ICPrevOutput=DiscIntNeverNeededParam  ICPrevScaledInput=DiscIntNeverNeededParam
  Multiply : Product  OutDataTypeStr=Inherit: Same as first input
  Saturation : Saturate  UpperLimit=max_i  LowerLimit=min_i
  ki : Constant  Value=ki  OutDataTypeStr=single
  i_out : Outport  VectorParamsAs1DForOutWhenUnconnected=off
  wires:
  err/1 -> Multiply/2
  Multiply/1 -> Discrete-Time Integrator/1
  reset/1 -> Discrete-Time Integrator/2
  Constant/1 -> Discrete-Time Integrator/3
  Discrete-Time Integrator/1 -> Saturation/1
  Saturation/1 -> i_out/1
  ki/1 -> Multiply/1

== system our_ch47/Subsystem/直升机3 PID control/位置控制器/侧向速度控制器/PID_Controller/P_Control ==
  err : Inport
  Multiply : Product  OutDataTypeStr=Inherit: Same as first input
  kp : Constant  Value=kp  OutDataTypeStr=single
  p_out : Outport  VectorParamsAs1DForOutWhenUnconnected=off
  wires:
  err/1 -> Multiply/2
  kp/1 -> Multiply/1
  Multiply/1 -> p_out/1

== system our_ch47/Subsystem/直升机3 PID control/位置控制器/前向位置控制器/前向位置控制器/PID_Controller ==
  err : Inport
  reset : Inport  Port=2
  Add : Sum
  I_Control : Subsystem  mask{ki=PID_Param1.Ki_x, max_i=1, min_i=-1}
  P_Control : Subsystem  mask{kp=PID_Param1.Kp_x}
  u : Outport  VectorParamsAs1DForOutWhenUnconnected=off
  wires:
  Add/1 -> u/1
  I_Control/1(i_out) -> Add/2
  P_Control/1(p_out) -> Add/1
  reset/1 -> I_Control/2(reset)
  err/1 -> I_Control/1(err), P_Control/1(err)

== system our_ch47/Subsystem/直升机3 PID control/位置控制器/前向速度控制器/PID_Controller/I_Control ==
  err : Inport
  reset : Inport  Port=2
  Constant : Constant  Value=0  OutDataTypeStr=single
  Discrete-Time Integrator : DiscreteIntegrator  ExternalReset=level  InitialConditionSource=external  SampleTime=-1  ICPrevOutput=DiscIntNeverNeededParam  ICPrevScaledInput=DiscIntNeverNeededParam
  Multiply : Product  OutDataTypeStr=Inherit: Same as first input
  Saturation : Saturate  UpperLimit=max_i  LowerLimit=min_i
  ki : Constant  Value=ki  OutDataTypeStr=single
  i_out : Outport  VectorParamsAs1DForOutWhenUnconnected=off
  wires:
  ki/1 -> Multiply/1
  Saturation/1 -> i_out/1
  Discrete-Time Integrator/1 -> Saturation/1
  Constant/1 -> Discrete-Time Integrator/3
  reset/1 -> Discrete-Time Integrator/2
  Multiply/1 -> Discrete-Time Integrator/1
  err/1 -> Multiply/2

== system our_ch47/Subsystem/直升机3 PID control/位置控制器/前向速度控制器/PID_Controller/P_Control ==
  err : Inport
  Multiply : Product  OutDataTypeStr=Inherit: Same as first input
  kp : Constant  Value=kp  OutDataTypeStr=single
  p_out : Outport  VectorParamsAs1DForOutWhenUnconnected=off
  wires:
  Multiply/1 -> p_out/1
  kp/1 -> Multiply/1
  err/1 -> Multiply/2

== system our_ch47/Subsystem/直升机3 PID control/位置控制器/垂向速度控制器/PID_Controller/I_Control ==
  err : Inport
  reset : Inport  Port=2
  Constant : Constant  Value=0  OutDataTypeStr=single
  Discrete-Time Integrator : DiscreteIntegrator  ExternalReset=level  InitialConditionSource=external  SampleTime=-1  ICPrevOutput=DiscIntNeverNeededParam  ICPrevScaledInput=DiscIntNeverNeededParam
  Multiply : Product  OutDataTypeStr=Inherit: Same as first input
  Saturation : Saturate  UpperLimit=max_i  LowerLimit=min_i
  ki : Constant  Value=ki  OutDataTypeStr=single
  i_out : Outport  VectorParamsAs1DForOutWhenUnconnected=off
  wires:
  ki/1 -> Multiply/1
  Saturation/1 -> i_out/1
  Discrete-Time Integrator/1 -> Saturation/1
  Constant/1 -> Discrete-Time Integrator/3
  reset/1 -> Discrete-Time Integrator/2
  Multiply/1 -> Discrete-Time Integrator/1
  err/1 -> Multiply/2

== system our_ch47/Subsystem/直升机3 PID control/位置控制器/垂向速度控制器/PID_Controller/P_Control ==
  err : Inport
  Multiply : Product  OutDataTypeStr=Inherit: Same as first input
  kp : Constant  Value=kp  OutDataTypeStr=single
  p_out : Outport  VectorParamsAs1DForOutWhenUnconnected=off
  wires:
  Multiply/1 -> p_out/1
  kp/1 -> Multiply/1
  err/1 -> Multiply/2

== system our_ch47/Subsystem/直升机3 PID control/位置控制器/高度控制器/高度控制器H-A/PID_Controller ==
  err : Inport
  reset : Inport  Port=2
  Add : Sum
  I_Control : Subsystem  mask{ki=PID_Param1.Ki_Hight, max_i=1, min_i=-1}
  P_Control : Subsystem  mask{kp=PID_Param1.Kp_Hight}
  u : Outport  VectorParamsAs1DForOutWhenUnconnected=off
  wires:
  Add/1 -> u/1
  I_Control/1(i_out) -> Add/2
  P_Control/1(p_out) -> Add/1
  reset/1 -> I_Control/2(reset)
  err/1 -> I_Control/1(err), P_Control/1(err)

== system our_ch47/Subsystem/直升机3 PID control/姿态控制器/俯仰控制器H-A/AltitudeV_Controller/PID_Controller ==
  err : Inport
  Add : Sum
  I_Control : Subsystem  mask{ki=PID_Param1.Ki_pitchrate, max_i=0.3, min_i=-0.3}
  P_Control : Subsystem  mask{kp=PID_Param1.Kp_pitchrate}
  u : Outport  VectorParamsAs1DForOutWhenUnconnected=off
  wires:
  Add/1 -> u/1
  I_Control/1(i_out) -> Add/2
  P_Control/1(p_out) -> Add/1
  err/1 -> I_Control/1(err), P_Control/1(err)

== system our_ch47/Subsystem/直升机3 PID control/姿态控制器/俯仰控制器H-A/角度换/PID_Controller ==
  err : Inport
  Add : Sum
  I_Control : Subsystem  mask{ki=PID_Param1.Ki_pitch, max_i=0.3, min_i=-0.3}
  P_Control : Subsystem  mask{kp=PID_Param1.Kp_pitch}
  u : Outport  VectorParamsAs1DForOutWhenUnconnected=off
  wires:
  Add/1 -> u/1
  I_Control/1(i_out) -> Add/2
  P_Control/1(p_out) -> Add/1
  err/1 -> I_Control/1(err), P_Control/1(err)

== system our_ch47/Subsystem/直升机3 PID control/姿态控制器/滚转控制器H-A/AltitudeV_Controller/PID_Controller ==
  err : Inport
  reset : Inport  Port=2
  Add : Sum
  I_Control : Subsystem  mask{ki=PID_Param1.Ki_rollrate, max_i=0.3, min_i=-0.3}
  P_Control : Subsystem  mask{kp=PID_Param1.Kp_rollrate}
  u : Outport  VectorParamsAs1DForOutWhenUnconnected=off
  wires:
  Add/1 -> u/1
  I_Control/1(i_out) -> Add/2  "i_out"
  P_Control/1(p_out) -> Add/1  "p_out"
  reset/1 -> I_Control/2(reset)
  err/1 -> I_Control/1(err), P_Control/1(err)

== system our_ch47/Subsystem/直升机3 PID control/姿态控制器/滚转控制器H-A/Altitude_Controller/PID_Controller ==
  err : Inport
  Add : Sum
  Constant : Constant  Value=0
  I_Control : Subsystem  mask{ki=PID_Param1.Ki_roll, max_i=0.3, min_i=-0.3}
  P_Control : Subsystem  mask{kp=PID_Param1.Kp_roll}
  u : Outport  VectorParamsAs1DForOutWhenUnconnected=off
  wires:
  Constant/1 -> I_Control/2(reset)
  Add/1 -> u/1
  I_Control/1(i_out) -> Add/2
  P_Control/1(p_out) -> Add/1
  err/1 -> I_Control/1(err), P_Control/1(err)

== system our_ch47/Subsystem/直升机3 PID control/姿态控制器/航向控制器H-A/AltitudeV_Controller/Controller ==
  err : Inport
  reset : Inport  Port=2
  Add : Sum
  I_Control : Subsystem  mask{ki=PID_Param1.Ki_yawrate, max_i=0.3, min_i=-0.3}
  P_Control : Subsystem  mask{kp=PID_Param1.Kp_yawrate}
  u : Outport  VectorParamsAs1DForOutWhenUnconnected=off
  wires:
  Add/1 -> u/1
  I_Control/1(i_out) -> Add/2
  P_Control/1(p_out) -> Add/1
  reset/1 -> I_Control/2(reset)
  err/1 -> I_Control/1(err), P_Control/1(err)

== system our_ch47/Subsystem/直升机3 PID control/姿态控制器/航向控制器H-A/Altitude_Controller/Controller ==
  err : Inport
  reset : Inport  Port=2
  Add : Sum
  I_Control : Subsystem  mask{ki=PID_Param1.Ki_yaw, max_i=5, min_i=-5}
  P_Control : Subsystem  mask{kp=PID_Param1.Kp_yaw}
  u : Outport  VectorParamsAs1DForOutWhenUnconnected=off
  wires:
  Add/1 -> u/1
  I_Control/1(i_out) -> Add/2
  P_Control/1(p_out) -> Add/1
  reset/1 -> I_Control/2(reset)
  err/1 -> I_Control/1(err), P_Control/1(err)

== system our_ch47/Subsystem/直升机4 PID control/位置控制器/侧向位置控制器/侧向位置控制器/PID_Controller ==
  err : Inport
  reset : Inport  Port=2
  Add : Sum
  I_Control : Subsystem  mask{ki=PID_Param1.Ki_y, max_i=1, min_i=-1}
  P_Control : Subsystem  mask{kp=PID_Param1.Kp_y}
  u : Outport  VectorParamsAs1DForOutWhenUnconnected=off
  wires:
  Add/1 -> u/1
  I_Control/1(i_out) -> Add/2
  P_Control/1(p_out) -> Add/1
  reset/1 -> I_Control/2(reset)
  err/1 -> I_Control/1(err), P_Control/1(err)

== system our_ch47/Subsystem/直升机4 PID control/位置控制器/侧向速度控制器/PID_Controller/I_Control ==
  err : Inport
  reset : Inport  Port=2
  Constant : Constant  Value=0  OutDataTypeStr=single
  Discrete-Time Integrator : DiscreteIntegrator  ExternalReset=level  InitialConditionSource=external  SampleTime=-1  ICPrevOutput=DiscIntNeverNeededParam  ICPrevScaledInput=DiscIntNeverNeededParam
  Multiply : Product  OutDataTypeStr=Inherit: Same as first input
  Saturation : Saturate  UpperLimit=max_i  LowerLimit=min_i
  ki : Constant  Value=ki  OutDataTypeStr=single
  i_out : Outport  VectorParamsAs1DForOutWhenUnconnected=off
  wires:
  ki/1 -> Multiply/1
  Saturation/1 -> i_out/1
  Discrete-Time Integrator/1 -> Saturation/1
  Constant/1 -> Discrete-Time Integrator/3
  reset/1 -> Discrete-Time Integrator/2
  Multiply/1 -> Discrete-Time Integrator/1
  err/1 -> Multiply/2

== system our_ch47/Subsystem/直升机4 PID control/位置控制器/侧向速度控制器/PID_Controller/P_Control ==
  err : Inport
  Multiply : Product  OutDataTypeStr=Inherit: Same as first input
  kp : Constant  Value=kp  OutDataTypeStr=single
  p_out : Outport  VectorParamsAs1DForOutWhenUnconnected=off
  wires:
  Multiply/1 -> p_out/1
  kp/1 -> Multiply/1
  err/1 -> Multiply/2

== system our_ch47/Subsystem/直升机4 PID control/位置控制器/前向位置控制器/前向位置控制器/PID_Controller ==
  err : Inport
  reset : Inport  Port=2
  Add : Sum
  I_Control : Subsystem  mask{ki=PID_Param1.Ki_x, max_i=1, min_i=-1}
  P_Control : Subsystem  mask{kp=PID_Param1.Kp_x}
  u : Outport  VectorParamsAs1DForOutWhenUnconnected=off
  wires:
  err/1 -> P_Control/1(err), I_Control/1(err)
  reset/1 -> I_Control/2(reset)
  P_Control/1(p_out) -> Add/1
  I_Control/1(i_out) -> Add/2
  Add/1 -> u/1

== system our_ch47/Subsystem/直升机4 PID control/位置控制器/前向速度控制器/PID_Controller/I_Control ==
  err : Inport
  reset : Inport  Port=2
  Constant : Constant  Value=0  OutDataTypeStr=single
  Discrete-Time Integrator : DiscreteIntegrator  ExternalReset=level  InitialConditionSource=external  SampleTime=-1  ICPrevOutput=DiscIntNeverNeededParam  ICPrevScaledInput=DiscIntNeverNeededParam
  Multiply : Product  OutDataTypeStr=Inherit: Same as first input
  Saturation : Saturate  UpperLimit=max_i  LowerLimit=min_i
  ki : Constant  Value=ki  OutDataTypeStr=single
  i_out : Outport  VectorParamsAs1DForOutWhenUnconnected=off
  wires:
  err/1 -> Multiply/2
  Multiply/1 -> Discrete-Time Integrator/1
  reset/1 -> Discrete-Time Integrator/2
  Constant/1 -> Discrete-Time Integrator/3
  Discrete-Time Integrator/1 -> Saturation/1
  Saturation/1 -> i_out/1
  ki/1 -> Multiply/1

== system our_ch47/Subsystem/直升机4 PID control/位置控制器/前向速度控制器/PID_Controller/P_Control ==
  err : Inport
  Multiply : Product  OutDataTypeStr=Inherit: Same as first input
  kp : Constant  Value=kp  OutDataTypeStr=single
  p_out : Outport  VectorParamsAs1DForOutWhenUnconnected=off
  wires:
  err/1 -> Multiply/2
  kp/1 -> Multiply/1
  Multiply/1 -> p_out/1

== system our_ch47/Subsystem/直升机4 PID control/位置控制器/垂向速度控制器/PID_Controller/I_Control ==
  err : Inport
  reset : Inport  Port=2
  Constant : Constant  Value=0  OutDataTypeStr=single
  Discrete-Time Integrator : DiscreteIntegrator  ExternalReset=level  InitialConditionSource=external  SampleTime=-1  ICPrevOutput=DiscIntNeverNeededParam  ICPrevScaledInput=DiscIntNeverNeededParam
  Multiply : Product  OutDataTypeStr=Inherit: Same as first input
  Saturation : Saturate  UpperLimit=max_i  LowerLimit=min_i
  ki : Constant  Value=ki  OutDataTypeStr=single
  i_out : Outport  VectorParamsAs1DForOutWhenUnconnected=off
  wires:
  err/1 -> Multiply/2
  Multiply/1 -> Discrete-Time Integrator/1
  reset/1 -> Discrete-Time Integrator/2
  Constant/1 -> Discrete-Time Integrator/3
  Discrete-Time Integrator/1 -> Saturation/1
  Saturation/1 -> i_out/1
  ki/1 -> Multiply/1

== system our_ch47/Subsystem/直升机4 PID control/位置控制器/垂向速度控制器/PID_Controller/P_Control ==
  err : Inport
  Multiply : Product  OutDataTypeStr=Inherit: Same as first input
  kp : Constant  Value=kp  OutDataTypeStr=single
  p_out : Outport  VectorParamsAs1DForOutWhenUnconnected=off
  wires:
  err/1 -> Multiply/2
  kp/1 -> Multiply/1
  Multiply/1 -> p_out/1

== system our_ch47/Subsystem/直升机4 PID control/位置控制器/高度控制器/高度控制器H-A/PID_Controller ==
  err : Inport
  reset : Inport  Port=2
  Add : Sum
  I_Control : Subsystem  mask{ki=PID_Param1.Ki_Hight, max_i=1, min_i=-1}
  P_Control : Subsystem  mask{kp=PID_Param1.Kp_Hight}
  u : Outport  VectorParamsAs1DForOutWhenUnconnected=off
  wires:
  err/1 -> P_Control/1(err), I_Control/1(err)
  reset/1 -> I_Control/2(reset)
  P_Control/1(p_out) -> Add/1
  I_Control/1(i_out) -> Add/2
  Add/1 -> u/1

== system our_ch47/Subsystem/直升机4 PID control/姿态控制器/俯仰控制器H-A/AltitudeV_Controller/PID_Controller ==
  err : Inport
  Add : Sum
  I_Control : Subsystem  mask{ki=PID_Param1.Ki_pitchrate, max_i=0.3, min_i=-0.3}
  P_Control : Subsystem  mask{kp=PID_Param1.Kp_pitchrate}
  u : Outport  VectorParamsAs1DForOutWhenUnconnected=off
  wires:
  err/1 -> P_Control/1(err), I_Control/1(err)
  P_Control/1(p_out) -> Add/1
  I_Control/1(i_out) -> Add/2
  Add/1 -> u/1

== system our_ch47/Subsystem/直升机4 PID control/姿态控制器/俯仰控制器H-A/角度换/PID_Controller ==
  err : Inport
  Add : Sum
  I_Control : Subsystem  mask{ki=PID_Param1.Ki_pitch, max_i=0.3, min_i=-0.3}
  P_Control : Subsystem  mask{kp=PID_Param1.Kp_pitch}
  u : Outport  VectorParamsAs1DForOutWhenUnconnected=off
  wires:
  err/1 -> P_Control/1(err), I_Control/1(err)
  P_Control/1(p_out) -> Add/1
  I_Control/1(i_out) -> Add/2
  Add/1 -> u/1

== system our_ch47/Subsystem/直升机4 PID control/姿态控制器/滚转控制器H-A/AltitudeV_Controller/PID_Controller ==
  err : Inport
  reset : Inport  Port=2
  Add : Sum
  I_Control : Subsystem  mask{ki=PID_Param1.Ki_rollrate, max_i=0.3, min_i=-0.3}
  P_Control : Subsystem  mask{kp=PID_Param1.Kp_rollrate}
  u : Outport  VectorParamsAs1DForOutWhenUnconnected=off
  wires:
  err/1 -> P_Control/1(err), I_Control/1(err)
  reset/1 -> I_Control/2(reset)
  P_Control/1(p_out) -> Add/1  "p_out"
  I_Control/1(i_out) -> Add/2  "i_out"
  Add/1 -> u/1

== system our_ch47/Subsystem/直升机4 PID control/姿态控制器/滚转控制器H-A/Altitude_Controller/PID_Controller ==
  err : Inport
  Add : Sum
  Constant : Constant  Value=0
  I_Control : Subsystem  mask{ki=PID_Param1.Ki_roll, max_i=0.3, min_i=-0.3}
  P_Control : Subsystem  mask{kp=PID_Param1.Kp_roll}
  u : Outport  VectorParamsAs1DForOutWhenUnconnected=off
  wires:
  err/1 -> P_Control/1(err), I_Control/1(err)
  P_Control/1(p_out) -> Add/1
  I_Control/1(i_out) -> Add/2
  Add/1 -> u/1
  Constant/1 -> I_Control/2(reset)

== system our_ch47/Subsystem/直升机4 PID control/姿态控制器/航向控制器H-A/AltitudeV_Controller/Controller ==
  err : Inport
  reset : Inport  Port=2
  Add : Sum
  I_Control : Subsystem  mask{ki=PID_Param1.Ki_yawrate, max_i=0.3, min_i=-0.3}
  P_Control : Subsystem  mask{kp=PID_Param1.Kp_yawrate}
  u : Outport  VectorParamsAs1DForOutWhenUnconnected=off
  wires:
  err/1 -> P_Control/1(err), I_Control/1(err)
  reset/1 -> I_Control/2(reset)
  P_Control/1(p_out) -> Add/1
  I_Control/1(i_out) -> Add/2
  Add/1 -> u/1

== system our_ch47/Subsystem/直升机4 PID control/姿态控制器/航向控制器H-A/Altitude_Controller/Controller ==
  err : Inport
  reset : Inport  Port=2
  Add : Sum
  I_Control : Subsystem  mask{ki=PID_Param1.Ki_yaw, max_i=5, min_i=-5}
  P_Control : Subsystem  mask{kp=PID_Param1.Kp_yaw}
  u : Outport  VectorParamsAs1DForOutWhenUnconnected=off
  wires:
  err/1 -> P_Control/1(err), I_Control/1(err)
  reset/1 -> I_Control/2(reset)
  P_Control/1(p_out) -> Add/1
  I_Control/1(i_out) -> Add/2
  Add/1 -> u/1

== system our_ch47/Subsystem/直升机1 PID control/位置控制器/侧向位置控制器/侧向位置控制器/PID_Controller/I_Control ==
  err : Inport
  reset : Inport  Port=2
  Constant : Constant  Value=0  OutDataTypeStr=single
  Discrete-Time Integrator : DiscreteIntegrator  ExternalReset=level  InitialConditionSource=external  SampleTime=-1  ICPrevOutput=DiscIntNeverNeededParam  ICPrevScaledInput=DiscIntNeverNeededParam
  Multiply : Product  OutDataTypeStr=Inherit: Same as first input
  Saturation : Saturate  UpperLimit=max_i  LowerLimit=min_i
  ki : Constant  Value=ki  OutDataTypeStr=single
  i_out : Outport  VectorParamsAs1DForOutWhenUnconnected=off
  wires:
  ki/1 -> Multiply/1
  Saturation/1 -> i_out/1
  Discrete-Time Integrator/1 -> Saturation/1
  Constant/1 -> Discrete-Time Integrator/3
  reset/1 -> Discrete-Time Integrator/2
  Multiply/1 -> Discrete-Time Integrator/1
  err/1 -> Multiply/2

== system our_ch47/Subsystem/直升机1 PID control/位置控制器/侧向位置控制器/侧向位置控制器/PID_Controller/P_Control ==
  err : Inport
  Multiply : Product  OutDataTypeStr=Inherit: Same as first input
  kp : Constant  Value=kp  OutDataTypeStr=single
  p_out : Outport  VectorParamsAs1DForOutWhenUnconnected=off
  wires:
  Multiply/1 -> p_out/1
  kp/1 -> Multiply/1
  err/1 -> Multiply/2

== system our_ch47/Subsystem/直升机1 PID control/位置控制器/前向位置控制器/前向位置控制器/PID_Controller/I_Control ==
  err : Inport
  reset : Inport  Port=2
  Constant : Constant  Value=0  OutDataTypeStr=single
  Discrete-Time Integrator : DiscreteIntegrator  ExternalReset=level  InitialConditionSource=external  SampleTime=-1  ICPrevOutput=DiscIntNeverNeededParam  ICPrevScaledInput=DiscIntNeverNeededParam
  Multiply : Product  OutDataTypeStr=Inherit: Same as first input
  Saturation : Saturate  UpperLimit=max_i  LowerLimit=min_i
  ki : Constant  Value=ki  OutDataTypeStr=single
  i_out : Outport  VectorParamsAs1DForOutWhenUnconnected=off
  wires:
  err/1 -> Multiply/2
  Multiply/1 -> Discrete-Time Integrator/1
  reset/1 -> Discrete-Time Integrator/2
  Constant/1 -> Discrete-Time Integrator/3
  Discrete-Time Integrator/1 -> Saturation/1
  Saturation/1 -> i_out/1
  ki/1 -> Multiply/1

== system our_ch47/Subsystem/直升机1 PID control/位置控制器/前向位置控制器/前向位置控制器/PID_Controller/P_Control ==
  err : Inport
  Multiply : Product  OutDataTypeStr=Inherit: Same as first input
  kp : Constant  Value=kp  OutDataTypeStr=single
  p_out : Outport  VectorParamsAs1DForOutWhenUnconnected=off
  wires:
  err/1 -> Multiply/2
  kp/1 -> Multiply/1
  Multiply/1 -> p_out/1

== system our_ch47/Subsystem/直升机1 PID control/位置控制器/高度控制器/高度控制器H-A/PID_Controller/I_Control ==
  err : Inport
  reset : Inport  Port=2
  Constant : Constant  Value=0  OutDataTypeStr=single
  Discrete-Time Integrator : DiscreteIntegrator  ExternalReset=level  InitialConditionSource=external  SampleTime=-1  ICPrevOutput=DiscIntNeverNeededParam  ICPrevScaledInput=DiscIntNeverNeededParam
  Multiply : Product  OutDataTypeStr=Inherit: Same as first input
  Saturation : Saturate  UpperLimit=max_i  LowerLimit=min_i
  ki : Constant  Value=ki  OutDataTypeStr=single
  i_out : Outport  VectorParamsAs1DForOutWhenUnconnected=off
  wires:
  err/1 -> Multiply/2
  Multiply/1 -> Discrete-Time Integrator/1
  reset/1 -> Discrete-Time Integrator/2
  Constant/1 -> Discrete-Time Integrator/3
  Discrete-Time Integrator/1 -> Saturation/1
  Saturation/1 -> i_out/1
  ki/1 -> Multiply/1

== system our_ch47/Subsystem/直升机1 PID control/位置控制器/高度控制器/高度控制器H-A/PID_Controller/P_Control ==
  err : Inport
  Multiply : Product  OutDataTypeStr=Inherit: Same as first input
  kp : Constant  Value=kp  OutDataTypeStr=single
  p_out : Outport  VectorParamsAs1DForOutWhenUnconnected=off
  wires:
  err/1 -> Multiply/2
  kp/1 -> Multiply/1
  Multiply/1 -> p_out/1

== system our_ch47/Subsystem/直升机1 PID control/姿态控制器/俯仰控制器H-A/AltitudeV_Controller/PID_Controller/I_Control ==
  err : Inport
  reset : Inport  Port=2
  Constant : Constant  Value=0  OutDataTypeStr=single
  Discrete-Time Integrator : DiscreteIntegrator  ExternalReset=level  InitialConditionSource=external  SampleTime=-1  ICPrevOutput=DiscIntNeverNeededParam  ICPrevScaledInput=DiscIntNeverNeededParam
  Multiply : Product  OutDataTypeStr=Inherit: Same as first input
  Saturation : Saturate  UpperLimit=max_i  LowerLimit=min_i
  ki : Constant  Value=ki  OutDataTypeStr=single
  i_out : Outport  VectorParamsAs1DForOutWhenUnconnected=off
  wires:
  err/1 -> Multiply/2
  Saturation/1 -> i_out/1
  ki/1 -> Multiply/1
  Discrete-Time Integrator/1 -> Saturation/1
  reset/1 -> Discrete-Time Integrator/2
  Multiply/1 -> Discrete-Time Integrator/1
  Constant/1 -> Discrete-Time Integrator/3
